simulink model "fsk_demod_1_noise"  (R2018a)
settings: Solver=VariableStepAuto  StartTime=0.0  StopTime=10.0  RelTol=1e-3
libraries: simulink x1, commrandsrc3 x1, commsynccomp2 x1
settings Model: Creator=hp  LastModifiedBy=hp

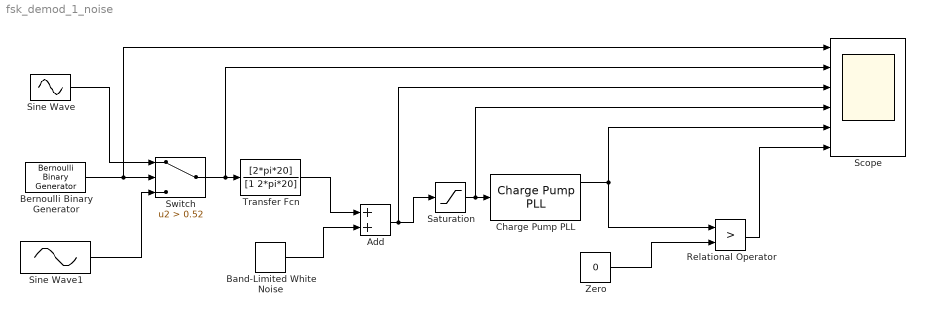
== system fsk_demod_1_noise ==
  Add : Sum
  Band-Limited White Noise : simulink/Sources/Band-Limited White Noise  Cov=[0.00002]  Ts=0.1  seed=[23341]
  Bernoulli Binary Generator : commrandsrc3/Bernoulli Binary Generator  ProbabilityOfZero=0.3  SeedSource=Auto  Seed=0  SampleTime=1  SamplesPerFrame=1  OutputDataType=double  SimulateUsing=Interpreted execution
  Charge Pump PLL : commsynccomp2/Charge Pump PLL  Fn=[2*pi*1]  Fd=[1 2*pi*1]  Kvco=1  Fc=10  Ph=0  Ac=1
      settings: SourceProductName=Communications System Toolbox  SourceProductBaseCode=CM
  Relational Operator : RelationalOperator  Operator=>  OutDataTypeStr=boolean  ZeroCross=off  RndMeth=Simplest
  Saturation : Saturate
  Scope : Scope  NumInputPorts=6
  Sine Wave : Sin  Frequency=2*pi*20  SampleTime=0.01
  Sine Wave1 : Sin  Frequency=2*pi*5  SampleTime=0.01
  Switch : Switch  Criteria=u2 > Threshold  Threshold=0.52
  Transfer Fcn : TransferFcn  Numerator=[2*pi*20]  Denominator=[1 2*pi*20]
  Zero : Constant  Value=0
  wires:
  Transfer Fcn/1 -> Add/1
  Sine Wave/1 -> Switch/1
  Relational Operator/1 -> Scope/6
  Switch/1 -> Scope/2, Transfer Fcn/1
  Add/1 -> Scope/3, Saturation/1
  Zero/1 -> Relational Operator/2
  Saturation/1 -> Scope/4, Charge Pump PLL/1
  Bernoulli Binary Generator/1 -> Scope/1, Switch/2
  Sine Wave1/1 -> Switch/3
  Charge Pump PLL/1 -> Relational Operator/1, Scope/5
  Band-Limited White Noise/1 -> Add/2
